simulink model "EX4_ex4"  (R2018b)
settings: Solver=VariableStepAuto  StartTime=0.0  StopTime=10.0  RelTol=1e-3
settings Model: Creator=吳俊逸  LastModifiedBy=吳俊逸

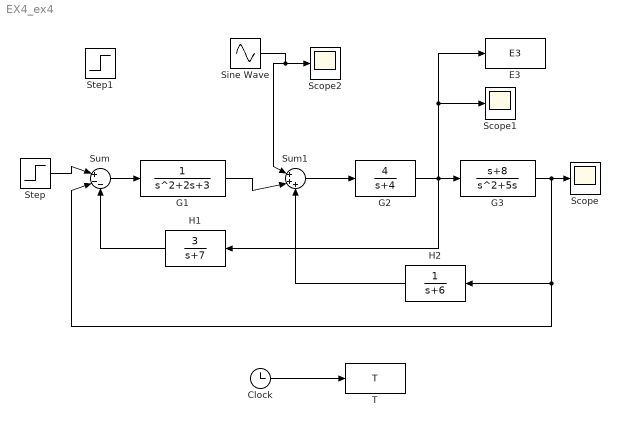
== system EX4_ex4 ==
  Clock : Clock
  "E3 " : ToWorkspace  VariableName=E3  SampleTime=-1
  G1 : TransferFcn  Denominator=[1 2 3]
  G2 : TransferFcn  Numerator=[4]  Denominator=[1 4]
  G3 : TransferFcn  Numerator=[1 8]  Denominator=[1 5 0]
  H1 : TransferFcn  Numerator=[3]  Denominator=[1 7]
  H2 : TransferFcn  Denominator=[1 6]
  Scope : Scope
  Scope1 : Scope
  Scope2 : Scope
  Sine Wave : Sin  Amplitude=0.2  Frequency=2  SampleTime=0
  Step : Step  Time=0  SampleTime=0
  Step1 : Step  Time=0  After=0.1  SampleTime=0
  Sum : Sum  Inputs=|+--
  Sum1 : Sum  Inputs=|+++
  "T " : ToWorkspace  VariableName=T  SampleTime=-1
  wires:
  Step/1 -> Sum/1
  Sum/1 -> G1/1
  H1/1 -> Sum/3
  G1/1 -> Sum1/2
  Sum1/1 -> G2/1
  G2/1 -> "E3 "/1, Scope1/1, G3/1, H1/1
  H2/1 -> Sum1/3
  G3/1 -> Scope/1, H2/1, Sum/2
  Clock/1 -> "T "/1
  Sine Wave/1 -> Sum1/1, Scope2/1
